simulink model "tutorial1"  (Simulink 2.20)
settings: Solver=ode5  StartTime=0.0  StopTime=tstop  FixedStep=tstep  MaxStep=tstep  RelTol=1e-3  AbsTol=1e-3
settings Model: SaveTime=off  SaveOutput=off  ConsistencyChecking=off  RTWPlaceOutputsASAP=off

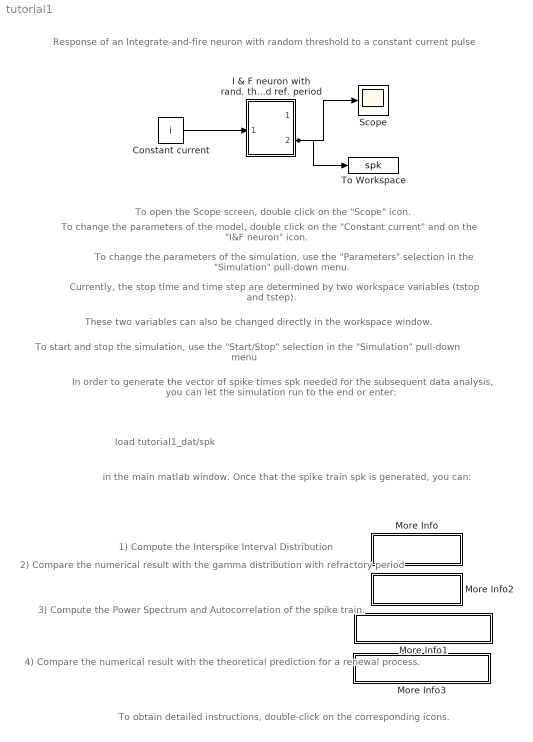
== system tutorial1 ==
  note: Response of an Integrate-and-fire neuron with
      | random threshold to a constant current pulse
  note: To start and stop the simulation, use the "Start/Stop"
      | selection in the "Simulation" pull-down menu
  note: To open the Scope screen, double click on the "Scope" icon.
  note: To change the parameters of the model, double click on the
      | "Constant current" and on the  "I&F neuron" icon.
  note: To change the parameters of the simulation, use the "Parameters"
      | selection in the "Simulation" pull-down menu.
  note: Currently, the stop time and time step are determined by two
      | workspace variables (tstop and tstep).
  note: These two variables can also be changed directly in the
      | workspace window.
  note: In order to generate the vector of spike times spk needed for the
      | subsequent data analysis, you can let the simulation run to the end
      | or enter:
  note: To obtain detailed instructions, double-click on the corresponding
      | icons.
  note: 1) Compute the Interspike Interval Distribution
  note: 2) Compare the numerical result with the
      | gamma distribution with refractory period
  note: 3) Compute the Power Spectrum and
      |  Autocorrelation of the spike train.
  note: 4) Compare the numerical result with the
      | theoretical prediction for a renewal process.
  note: load tutorial1_dat/spk
  note: in the main matlab window. Once that the spike train spk is generated,
      | you can:
  Constant current : Constant  Value=i  mask(constant current){@1=0.6}
      mask prompts: @1 "constant current value [nA]"
      mask help: Parameter
      mask init:
      | i = @1;
      mask Help: Provides a constant input current
  I & F neuron with rand. thres. and ref. period : Subsystem  mask(I&F g. thres., ref. per.){@1=tstep, @2=10, @3=5, @4=0.5, @5=5}
      mask prompts: @1 "time step [msec]"; @2 "mean threshold [mV]"; @3 "gamma distr. order"; @4 "Capacitance [nF]"; @5 "refractory period [msec]"
      mask help: Parameters
      mask init:
      | dt = @1; thres = @2; n = @3; C = @4; ref = @5; if (ref<dt) disp(' '); disp('Warning: refractory period cannot be smaller than time step.'); disp(' '); end;
      mask Help: For a detailled description of the model, please type 'help giandfr' in the main matlab window
      mask Display: disp('Vm \n\n spikes')
  More Info : Subsystem
      mask Display: disp('Numerical ISI')
  More Info1 : Subsystem
      mask Display: disp('Numerical PS and AC')
  More Info2 : Subsystem
      mask Display: disp('Theoretical ISI')
  More Info3 : Subsystem
      mask Display: disp('Theoretical PS and AC')
  Scope : Scope
      settings: TickLabels=on  TimeRange=500.000000  YMin=-2.000000  YMax=2.000000  SaveToWorkspace=off  SaveName=ScopeData
  To Workspace : ToWorkspace  VariableName=spk  SampleTime=0
      settings: Buffer=ceil(tstop/tstep)
  wires:
  Constant current/1 -> I & F neuron with rand. thres. and ref. period/1(in_1)
  I & F neuron with rand. thres. and ref. period/2(out_1) -> Scope/1, To Workspace/1

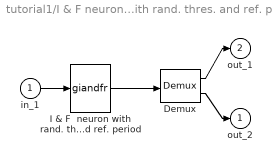
== system tutorial1/I & F neuron with rand. thres. and ref. period ==
  in_1 : Inport  Port=1  PortWidth=-1  SampleTime=-1
  Demux : Demux  Outputs=2
  I & F  neuron with rand. thres. and ref. period : S-Function  FunctionName=giandfr  Parameters=dt,thres,n,C,ref  PortCounts=[]  SFunctionModules=''
  out_2 : Outport  Port=1  InitialOutput=0
  out_1 : Outport  Port=2  InitialOutput=0
  wires:
  in_1/1 -> I & F  neuron with rand. thres. and ref. period/1
  Demux/2 -> out_2/1
  Demux/1 -> out_1/1
  I & F  neuron with rand. thres. and ref. period/1 -> Demux/1

== system tutorial1/More Info ==
  note: To compute the ISI distribution
      | corresponding to the spike train, enter
  note: isidist(spk,2,100,tstep).
  note: in the workspace window.
  note: The parameters are:
  note: spk = spike train generated by the simulation of the model.
  note: 2 = bin size in msec
  note: 100 = maximal isi in msec
  note: tstep = time step for the simulation

== system tutorial1/More Info1 ==
  note: To compute the power spectrum and
      | the autocorrelation of the spike train, enter
  note: psautospk(spk,tstep).
  note: tstep = time step for the simulation
  note: spk = spike train generated by the simulation of the model.
  note: The parameters are:

== system tutorial1/More Info2 ==
  note: tstep = time step for the simulation
  note: 100 = maximal isi in msec
  note: 2 = bin size in msec
  note: 5 = refractory period (msec)
  note: 0.6 = constant injected current (nA)
  note: 5 = order of the gamma distribution determining the
      |       noise in the threshold.
  note: 10 = mean spike threshold (mV)
  note: 0.5 = Capacity of the model cell (nF)
  note: The parameters are:
  note: To compare the theoretical ISI distribution  with the
      | previously obtained numerical ISI distribution, enter
  note: gfitheor(0.5,10,5,0.6,5,2,100,tstep).
  note: hold on
  note: in the workspace window.

== system tutorial1/More Info3 ==
  note: To compare the theoretical power spectrum and autocorrelation
      | function with the previously obtained numerical power spectrum
      | and autocorrelation function, enter
  note: hold on
  note: 1024 = number of bins between 0 and the Nyquist frequency
  note: tstep = time step for the simulation
  note: 5 = order of the gamma distribution determining the
      |       noise in the threshold.
  note: 5 = refractory period (msec)
  note: 0.6 = constant injected current (nA)
  note: 10 = mean spike threshold (mV)
  note: 0.5 = Capacity of the model cell (nF)
  note: The parameters are:
  note: in the workspace window.
  note: gpstheor(0.5,10,0.6,5,5,tstep,1024)
  note: hold on
  note: subplot(2,1,1)
